simulink model "TV2016"  (Simulink 8.5)
settings: Solver=FixedStepDiscrete  StartTime=0.0  StopTime=inf  FixedStep=0.001  RelTol=1e-3
PreLoadFcn:
  | FSE_Parameters
values from neighbouring files (symbols this model uses):
  car_params = Simulink_Car_params    [TV2016_parameters.m]
  i_Diff = 15.47    [TV2016_parameters.m]
  Kp = 1    [TV2016_parameters.m]
  powerLimitControl = Simulink_el    [TV2016_parameters.m]
  settings = Simulink_Settings    [TV2016_parameters.m]
  SpdC_BCC = 0    [TV2016_parameters.m]
  Speed_Neg_sat = -21    [TV2016_parameters.m]
  Speed_Pos_sat = 21    [TV2016_parameters.m]
  speedEstimation = Simulink_speedEst    [TV2016_parameters.m]
  Tn_n = 0    [TV2016_parameters.m]
  tractionControl = Simulink_tc    [TV2016_parameters.m]
  Use_Joystick = 1    [TV2016_parameters.m]
  yawRateControl = Simulink_yawRate    [TV2016_parameters.m]
libraries: CarMaker4SL x174, simulink x27, simulink_extras x14
(part 3 of 5)

== system TV2016/CarMaker/Control_System /Control /Slip Rate Control  ==
  Ti_ref : Inport
  "States " : Inport  Port=2
  T_req : Inport  Port=3
  Bus Selector : BusSelector  OutputSignals=FL,FR,RL,RR
  Constant : Constant  Value=tractionControl.enable
  Index Vector : MultiPortSwitch  DataPortOrder=Zero-based contiguous  Inputs=2  zeroidx=on
  Mux18 : Mux
  SMC Traction Control : Subsystem  Commented=on
  Traction Controllers : Subsystem
  tcOutput : Scope
      settings: ShowLegends=on  YMin=0.1998305084745763  YMax=0.2840677966101695  SaveName=ScopeData31
  Ti_lim : Outport
  wires:
  "States "/1 -> Traction Controllers/1(states)
  Ti_ref/1 -> Traction Controllers/2(Ti_ref), Index Vector/2
  Index Vector/1 -> Ti_lim/1
  Constant/1 -> Index Vector/1
  T_req/1 -> Traction Controllers/3(T_requested)
  Traction Controllers/1(Ti_SR) -> Bus Selector/1, Index Vector/3
  Mux18/1 -> tcOutput/1
  Bus Selector/1 -> Mux18/1  "<FL>"
  Bus Selector/2 -> Mux18/2  "<FR>"
  Bus Selector/3 -> Mux18/3  "<RL>"
  Bus Selector/4 -> Mux18/4  "<RR>"

== system TV2016/CarMaker/Control_System /Control /Throttle / Brake Mapping ==
  "states " : Inport
  MATLAB Function : MATLAB Function  TreatAsAtomicUnit=on
  T_req : Outport
  wires:
  "states "/1 -> MATLAB Function/1(states)
  MATLAB Function/1(T_req) -> T_req/1

== system TV2016/CarMaker/Control_System /Control /Torque allocation  ==
  Mz_ref : Inport
  T_req : Inport  Port=2
  "States " : Inport  Port=3
  Bus Selector : BusSelector  OutputSignals=mmt_FL,mmt_FR,mmt_RL,mmt_RR
  Index Vector2 : MultiPortSwitch
  MATLAB Function : MATLAB Function  TreatAsAtomicUnit=on
  Mux18 : Mux
  Switch Case : SwitchCase  CaseConditions={1,2,3}
  Switch Case Action Subsystem : Subsystem  TreatAsAtomicUnit=on
  Switch Case Action Subsystem1 : Subsystem  TreatAsAtomicUnit=on
  Switch Case Action Subsystem2 : Subsystem  TreatAsAtomicUnit=on
  Torque Allocation : Subsystem
  maxmotortoruq : Scope
      settings: ShowLegends=on  YMin=0.1998305084745763  YMax=0.2840677966101695  SaveName=ScopeData44
  Ti_lim : Outport
  "Mz_error " : Outport  Port=2
  wires:
  "States "/1 -> MATLAB Function/1(states), Torque Allocation/2(states)
  Mz_ref/1 -> Torque Allocation/4(Mz_ref)
  Torque Allocation/2(Mz_error) -> "Mz_error "/1
  MATLAB Function/1(maxMotorTorque) -> Bus Selector/1, Torque Allocation/3(maxMotorTorque)
  Mux18/1 -> maxmotortoruq/1
  Bus Selector/1 -> Mux18/1  "<mmt_FL>"
  Bus Selector/2 -> Mux18/2  "<mmt_FR>"
  Bus Selector/3 -> Mux18/3  "<mmt_RL>"
  Bus Selector/4 -> Mux18/4  "<mmt_RR>"
  Switch Case/1 -> Switch Case Action Subsystem1/Action
  Switch Case/2 -> Switch Case Action Subsystem/Action
  Switch Case/3 -> Switch Case Action Subsystem2/Action
  ? -> Index Vector2/1, Switch Case/1
  T_req/1 -> Torque Allocation/1(T_req)
  Torque Allocation/1(Ti_lim) -> Ti_lim/1

== system TV2016/CarMaker/Control_System /Control /Yaw Rate Controller  ==
  States : Inport
  "Mz_error " : Inport  Port=2
  Discrete-Time Integrator2 : DiscreteIntegrator  InitialConditionSetting=State (most efficient)  SampleTime=-1
  Enable/disable : Constant  Value=yawRateControl.enable
  Gain : Gain  Gain=single(3.6)
  Gain1 : Gain  Gain=single(3.6)
  Gain2 : Gain  Gain=single(3.6)
  Kd lookup : Lookup_n-D  NumberOfTableDimensions=1  BreakpointsForDimension1="[0  yawRateControl.lookup_speed_end_kmh]"  Table="[yawRateControl.Kd_start  yawRateControl.Kd_end]*yawRateControl.Kd_scaling"  ExtrapMethod=Clip  UseLastTableValue=on  InternalRulePriority=Speed  RndMeth=Simplest  InputSameDT=on
  Ki lookup : Lookup_n-D  NumberOfTableDimensions=1  BreakpointsForDimension1="[0  yawRateControl.lookup_speed_end_kmh]"  Table="[yawRateControl.Ki_start  yawRateControl.Ki_end]*yawRateControl.Ki_scaling"  ExtrapMethod=Clip  UseLastTableValue=on  InternalRulePriority=Speed  RndMeth=Simplest  InputSameDT=on
  Kp Lookup : Lookup_n-D  NumberOfTableDimensions=1  BreakpointsForDimension1="[0  yawRateControl.lookup_speed_end_kmh]"  Table="[yawRateControl.Kp_start  yawRateControl.Kp_end]*yawRateControl.Kp_scaling"  ExtrapMethod=Clip  UseLastTableValue=on  InternalRulePriority=Speed  RndMeth=Simplest  InputSameDT=on
  Ksat : Constant  Value=yawRateControl.Ksat
  "Mzerror " : Scope
      settings: ShowLegends=on  YMin=333.5  YMax=341  SaveName=ScopeData30
  PI_Kp {1..4} (4 alike) : Scope
      PI_Kp 1 settings: ShowLegends=on  YMin=333.5  YMax=341  SaveName=ScopeData3
      PI_Kp 2 settings: ShowLegends=on  YMin=333.5  YMax=341
      PI_Kp 3 settings: ShowLegends=on  TimeRange=4  YMin=333.8411144578313  YMax=336.8411144578313  SaveName=ScopeData9
      PI_Kp 4 settings: ShowLegends=on  YMin=333.5  YMax=341  SaveName=ScopeData18
  Product{7..8,10..11} (4 alike) : Product
  Product3 : Product  OutDataTypeStr=single
  Saturation : Saturate  UpperLimit=yawRateControl.max_moment  LowerLimit=-yawRateControl.max_moment
  Sum2 : Sum  Inputs=+++  AccumDataTypeStr=single
  Sum3 : Sum  Inputs=|+-
  derivative : Scope
      settings: ShowLegends=on  YMin=333.5  YMax=341  SaveName=ScopeData28
  yawRateReference : MATLAB Function  TreatAsAtomicUnit=on
  "r_ref " : Outport
  r_lim : Outport  Port=2
  ay_max : Outport  Port=3
  Mz_ref : Outport  Port=4  OutDataTypeStr=single
  wires:
  States/1 -> yawRateReference/1(states)
  yawRateReference/4(r_ref) -> "r_ref "/1
  yawRateReference/5(r_lim) -> r_lim/1
  yawRateReference/6(ay_max) -> ay_max/1
  Product7/1 -> Sum2/2, PI_Kp 1/1
  Sum2/1 -> Product3/2
  Product8/1 -> Sum3/1
  Sum3/1 -> Discrete-Time Integrator2/1
  Discrete-Time Integrator2/1 -> PI_Kp 3/1, Sum2/3
  Product11/1 -> Sum3/2
  yawRateReference/1(r_der_error) -> Product10/2, PI_Kp 4/1
  Kd lookup/1 -> Product10/1
  Product10/1 -> Sum2/1, derivative/1
  Kp Lookup/1 -> Product7/1
  Ksat/1 -> Product11/1
  "Mz_error "/1 -> "Mzerror "/1, Product11/2
  Ki lookup/1 -> Product8/2
  yawRateReference/2(r_error) -> Product8/1, Product7/2, PI_Kp 2/1
  Product3/1 -> Saturation/1
  Saturation/1 -> Mz_ref/1
  Enable/disable/1 -> Product3/1
  Gain/1 -> Kp Lookup/1
  Gain2/1 -> Ki lookup/1
  yawRateReference/3(vx) -> Gain/1, Gain1/1, Gain2/1
  Gain1/1 -> Kd lookup/1

== system TV2016/CarMaker/IPG Vehicle/Brake/CreateBus Vhcl.Wheel.PT ==
  In : Inport
  BusCreator : BusCreator  Inputs=16
  Demux : Demux  Outputs=16
  Out : Outport
  wires:
  Demux/16 -> BusCreator/16  "Vhcl Wheel RR WhlBearing"
  Demux/15 -> BusCreator/15  "Vhcl Wheel RR Trq_T2W"
  Demux/14 -> BusCreator/14  "Vhcl Wheel RR Trq_BrakeReg_trg"
  Demux/13 -> BusCreator/13  "Vhcl Wheel RR Trq_Brake"
  Demux/12 -> BusCreator/12  "Vhcl Wheel RL WhlBearing"
  Demux/11 -> BusCreator/11  "Vhcl Wheel RL Trq_T2W"
  Demux/10 -> BusCreator/10  "Vhcl Wheel RL Trq_BrakeReg_trg"
  Demux/9 -> BusCreator/9  "Vhcl Wheel RL Trq_Brake"
  Demux/8 -> BusCreator/8  "Vhcl Wheel FR WhlBearing"
  Demux/7 -> BusCreator/7  "Vhcl Wheel FR Trq_T2W"
  Demux/6 -> BusCreator/6  "Vhcl Wheel FR Trq_BrakeReg_trg"
  Demux/5 -> BusCreator/5  "Vhcl Wheel FR Trq_Brake"
  Demux/4 -> BusCreator/4  "Vhcl Wheel FL WhlBearing"
  Demux/3 -> BusCreator/3  "Vhcl Wheel FL Trq_T2W"
  Demux/2 -> BusCreator/2  "Vhcl Wheel FL Trq_BrakeReg_trg"
  Demux/1 -> BusCreator/1  "Vhcl Wheel FL Trq_Brake"
  BusCreator/1 -> Out/1
  In/1 -> Demux/1

== system TV2016/CarMaker/IPG Vehicle/CarAndTrailer/CarAndTrailerUpd ==
  Sync_In : Inport
  Vhcl.Steering : Inport  Port=2
  Vhcl.Motion : Inport  Port=3
  Vhcl.PoI : Inport  Port=4
  Vhcl.Wheel.FL : Inport  Port=5
  Vhcl.Wheel.FR : Inport  Port=6
  Vhcl.Wheel.RL : Inport  Port=7
  Vhcl.Wheel.RR : Inport  Port=8
  Car.Hitch.FrcTrq : Inport  Port=9
  Vhcl.Fr1A : Inport  Port=10
  CarAndTrailerUpd : S-Function  FunctionName=CM_Sfun  Parameters='CarAndTrUpd'
  CreateBus Brake.IF.In : Subsystem
  Sync_Out : Outport
  Brake.IF.In : Outport  Port=2
  wires:
  Vhcl.Fr1A/1 -> CarAndTrailerUpd/10  "user vehicle only"
  Vhcl.Steering/1 -> CarAndTrailerUpd/2
  Vhcl.Motion/1 -> CarAndTrailerUpd/3
  Vhcl.PoI/1 -> CarAndTrailerUpd/4
  Vhcl.Wheel.FL/1 -> CarAndTrailerUpd/5
  Vhcl.Wheel.FR/1 -> CarAndTrailerUpd/6
  Car.Hitch.FrcTrq/1 -> CarAndTrailerUpd/9
  Vhcl.Wheel.RR/1 -> CarAndTrailerUpd/8
  Vhcl.Wheel.RL/1 -> CarAndTrailerUpd/7
  CarAndTrailerUpd/2 -> CreateBus Brake.IF.In/1(In)
  CreateBus Brake.IF.In/1(Out) -> Brake.IF.In/1
  CarAndTrailerUpd/1 -> Sync_Out/1
  Sync_In/1 -> CarAndTrailerUpd/1

== system TV2016/CarMaker/IPG Vehicle/CarAndTrailer/Forces ==
  Sync_In : Inport
  TireFL_In : Inport  Port=2
  TireFR_In : Inport  Port=3
  TireRL_In : Inport  Port=4
  TireRR_In : Inport  Port=5
  lSpring : Inport  Port=6
  vDamp : Inport  Port=7
  lStabi : Inport  Port=8
  lBuf : Inport  Port=9
  External Suspension Forces : Subsystem
  Tires : Subsystem
  Vehicle Forces : Subsystem
  Sync_Out : Outport
  Car.Virtual : Outport  Port=2
  Car.Aero : Outport  Port=3
  Car.Load : Outport  Port=4
  TireFL_Out : Outport  Port=5
  TireFR_Out : Outport  Port=6
  TireRL_Out : Outport  Port=7
  TireRR_Out : Outport  Port=8
  FSpring : Outport  Port=9
  FDamp : Outport  Port=10
  FStabi : Outport  Port=11
  FBuf : Outport  Port=12
  wires:
  External Suspension Forces/4(FBuf) -> FBuf/1
  lBuf/1 -> External Suspension Forces/5(lBuf)
  Tires/1(TireFL_Out) -> TireFL_Out/1
  Tires/4(TireRR_Out) -> TireRR_Out/1
  Tires/3(TireRL_Out) -> TireRL_Out/1
  Tires/2(TireFR_Out) -> TireFR_Out/1
  TireRR_In/1 -> Tires/4(TireRR_In)
  TireRL_In/1 -> Tires/3(TireRL_In)
  TireFR_In/1 -> Tires/2(TireFR_In)
  Sync_In/1 -> External Suspension Forces/1(Sync_In), Tires/5(Sync_In), Vehicle Forces/1(Sync_In)
  Vehicle Forces/1(Sync_Out) -> Sync_Out/1
  TireFL_In/1 -> Tires/1(TireFL_In)
  Vehicle Forces/2(Car.Virtual) -> Car.Virtual/1
  Vehicle Forces/3(Car.Aero) -> Car.Aero/1
  Vehicle Forces/4(Car.Load) -> Car.Load/1
  lSpring/1 -> External Suspension Forces/2(lSpring)
  External Suspension Forces/2(FDamp) -> FDamp/1
  vDamp/1 -> External Suspension Forces/3(vDamp)
  lStabi/1 -> External Suspension Forces/4(lStabi)
  External Suspension Forces/3(FStabi) -> FStabi/1
  External Suspension Forces/1(FSpring) -> FSpring/1

== system TV2016/CarMaker/IPG Vehicle/CarAndTrailer/Kinematics ==
  Sync_In : Inport
  Steer.IF : Inport  Port=2
  Kinematics : S-Function  FunctionName=CM_Sfun  Parameters='Kinematics'
  Sync_Out : Outport
  TireFL_In : Outport  Port=2
  TireFR_In : Outport  Port=3
  TireRL_In : Outport  Port=4
  TireRR_In : Outport  Port=5
  lSpring : Outport  Port=6
  vDamp : Outport  Port=7
  lStabi : Outport  Port=8
  lBuf : Outport  Port=9
  wires:
  Kinematics/9 -> lBuf/1
  Kinematics/8 -> lStabi/1
  Kinematics/2 -> TireFL_In/1
  Kinematics/3 -> TireFR_In/1
  Kinematics/4 -> TireRL_In/1
  Kinematics/5 -> TireRR_In/1
  Kinematics/6 -> lSpring/1
  Kinematics/7 -> vDamp/1
  Sync_In/1 -> Kinematics/1
  Kinematics/1 -> Sync_Out/1
  Steer.IF/1 -> Kinematics/2

== system TV2016/CarMaker/IPG Vehicle/CarAndTrailer/Kinetics ==
  Sync_In : Inport
  Car.Virtual : Inport  Port=2
  Car.Aero : Inport  Port=3
  Car.Load : Inport  Port=4
  TireFL.Out : Inport  Port=5
  TireFR.Out : Inport  Port=6
  TireRL.Out : Inport  Port=7
  TireRR.Out : Inport  Port=8
  FSpring : Inport  Port=9
  FDamp : Inport  Port=10
  FStabi : Inport  Port=11
  FBuf : Inport  Port=12
  Bus Creator : BusCreator
  Bus Creator1 : BusCreator  Inputs=12
  Bus Creator2 : BusCreator  Inputs=6
  Bus Creator3 : BusCreator  Inputs=6
  Bus Creator4 : BusCreator
  Demux : Demux  Outputs=12
  Demux1 : Demux  Outputs=6
  Demux2 : Demux  Outputs=6
  Demux3 : Demux
  Demux4 : Demux
  Kinetics : S-Function  FunctionName=CM_Sfun  Parameters='Kinetics'
  Sync_Out : Outport
  Trailer.Load : Outport  Port=2
  Car.Hitch : Outport  Port=3
  Car.Fr1 : Outport  Port=4
  Car.Trq_T2W : Outport  Port=5
  WheelCarrier.Misc : Outport  Port=6
  wires:
  FBuf/1 -> Kinetics/12
  Sync_In/1 -> Kinetics/1
  Kinetics/1 -> Sync_Out/1
  Car.Aero/1 -> Kinetics/3
  Car.Virtual/1 -> Kinetics/2
  Bus Creator1/1 -> Trailer.Load/1
  Demux/1 -> Bus Creator1/1  "Trailer Load_0 mass"
  Demux/2 -> Bus Creator1/2  "Trailer Load_0 tx"
  Demux/3 -> Bus Creator1/3  "Trailer Load_0 ty"
  Demux/4 -> Bus Creator1/4  "Trailer Load_0 tz"
  Kinetics/2 -> Demux/1
  Demux/5 -> Bus Creator1/5  "Trailer Load_1 mass"
  Demux/6 -> Bus Creator1/6  "Trailer Load_1 tx"
  Demux/7 -> Bus Creator1/7  "Trailer Load_1 ty"
  Demux/8 -> Bus Creator1/8  "Trailer Load_1 tz"
  Demux/9 -> Bus Creator1/9  "Trailer Load_2 mass"
  Demux/10 -> Bus Creator1/10  "Trailer Load_2 tx"
  Demux/11 -> Bus Creator1/11  "Trailer Load_2 ty"
  Demux/12 -> Bus Creator1/12  "Trailer Load_2 tz"
  Demux1/1 -> Bus Creator2/1  "Car Hitch tx"
  Demux1/2 -> Bus Creator2/2  "Car Hitch ty"
  Demux1/3 -> Bus Creator2/3  "Car Hitch tz"
  Demux1/4 -> Bus Creator2/4  "Car Hitch vx"
  Demux1/5 -> Bus Creator2/5  "Car Hitch vy"
  Demux1/6 -> Bus Creator2/6  "Car Hitch vz"
  Kinetics/3 -> Demux1/1
  Bus Creator2/1 -> Car.Hitch/1
  Demux2/1 -> Bus Creator3/1  "Car Fr1 rx"
  Demux2/2 -> Bus Creator3/2  "Car Fr1 ry"
  Demux2/3 -> Bus Creator3/3  "Car Fr1 rz"
  Demux2/4 -> Bus Creator3/4  "Car Fr1 rvx"
  Demux2/5 -> Bus Creator3/5  "Car Fr1 rvy"
  Demux2/6 -> Bus Creator3/6  "Car Fr1 rvz"
  Bus Creator3/1 -> Car.Fr1/1
  Kinetics/4 -> Demux2/1
  Car.Load/1 -> Kinetics/4
  Demux3/1 -> Bus Creator4/1  "car Susp FL GenInert2"
  Demux3/2 -> Bus Creator4/2  "car Susp FR GenInert2"
  Demux3/3 -> Bus Creator4/3  "car Susp FL GenFrc2"
  Demux3/4 -> Bus Creator4/4  "car Susp FR GenFrc2"
  Bus Creator4/1 -> WheelCarrier.Misc/1
  Bus Creator/1 -> Car.Trq_T2W/1
  Demux4/4 -> Bus Creator/4  "Car Trq_T2WRR"
  Demux4/3 -> Bus Creator/3  "Car Trq_T2WRL"
  Demux4/2 -> Bus Creator/2  "Car Trq_T2WFR"
  Demux4/1 -> Bus Creator/1  "Car Trq_T2WFL"
  TireFL.Out/1 -> Kinetics/5
  TireFR.Out/1 -> Kinetics/6
  TireRL.Out/1 -> Kinetics/7
  TireRR.Out/1 -> Kinetics/8
  FSpring/1 -> Kinetics/9
  FDamp/1 -> Kinetics/10
  FStabi/1 -> Kinetics/11
  Kinetics/6 -> Demux3/1
  Kinetics/5 -> Demux4/1

== system TV2016/CarMaker/IPG Vehicle/CarAndTrailer/Steering ==
  note: When replacing the entire steering system,
      | be sure to add '-disablesteering' to the command line arguments
      | in the CarMaker Model Configuration block.
  Sync_In : Inport
  VhclCtrl.Steering : Inport  Port=2
  Bus Creator1 : BusCreator  Inputs=16
  Bus Creator2 : BusCreator
  Demux : Demux  Outputs=20
  Steering : S-Function  FunctionName=CM_Sfun  Parameters='Steering'
  Terminator : Terminator
  Sync_Out : Outport
  Steer.IF : Outport  Port=2
  wires:
  Bus Creator1/1 -> Steer.IF/1
  Steering/2 -> Demux/1
  Demux/8 -> Bus Creator1/8  "Steering IF AssistTrqPin"
  Demux/7 -> Bus Creator1/7  "Steering IF AssistTrqCol"
  Demux/6 -> Bus Creator1/6  "Steering IF AssistFrc"
  Demux/20 -> Bus Creator2/4  "Steering IF R Inert"
  Demux/17 -> Bus Creator2/1  "Steering IF L Frc"
  Demux/18 -> Bus Creator2/2  "Steering IF L Inert"
  Demux/19 -> Bus Creator2/3  "Steering IF R Frc"
  Bus Creator2/1 -> Terminator/1  "Steer IF (in)"
  Demux/16 -> Bus Creator1/16  "Steering IF R iSteer2q"
  Demux/9 -> Bus Creator1/9  "Steering IF L q"
  Demux/10 -> Bus Creator1/10  "Steering IF L qp"
  Demux/11 -> Bus Creator1/11  "Steering IF L qpp"
  Demux/12 -> Bus Creator1/12  "Steering IF L iSteer2q"
  Demux/13 -> Bus Creator1/13  "Steering IF R q"
  Demux/14 -> Bus Creator1/14  "Steering IF R qp"
  Demux/15 -> Bus Creator1/15  "Steering IF R qpp"
  VhclCtrl.Steering/1 -> Steering/2
  Steering/1 -> Sync_Out/1
  Sync_In/1 -> Steering/1
  Demux/1 -> Bus Creator1/1  "Steering IF Ang"
  Demux/2 -> Bus Creator1/2  "Steering IF AngVel"
  Demux/3 -> Bus Creator1/3  "Steering IF AngAcc"
  Demux/4 -> Bus Creator1/4  "Steering IF Trq"
  Demux/5 -> Bus Creator1/5  "Steering IF TrqStatic"

== system TV2016/CarMaker/IPG Vehicle/CarAndTrailer/Trailer ==
  Sync_In : Inport
  Trailer.Load : Inport  Port=2
  Car.Hitch : Inport  Port=3
  Car.Fr1 : Inport  Port=4
  Car.Trq_T2W : Inport  Port=5
  WheelCarrier.Misc : Inport  Port=6
  CreateBus Car.Hitch.FrcTrq : Subsystem
  CreateBus Vhcl.Motion : Subsystem
  CreateBus Vhcl.PoI : Subsystem
  CreateBus Vhcl.Steering : Subsystem
  CreateBus Vhcl.Wheel.FL : Subsystem
  CreateBus Vhcl.Wheel.FR : Subsystem
  CreateBus Vhcl.Wheel.RL : Subsystem
  CreateBus Vhcl.Wheel.RR : Subsystem
  Trailer : S-Function  FunctionName=CM_Sfun  Parameters='Trailer'
  Sync_Out : Outport
  Vhcl.Steering : Outport  Port=2
  Vhcl.Motion : Outport  Port=3
  Vhcl.PoI : Outport  Port=4
  Vhcl.Wheel.FL : Outport  Port=5
  Vhcl.Wheel.FR : Outport  Port=6
  Vhcl.Wheel.RL : Outport  Port=7
  Vhcl.Wheel.RR : Outport  Port=8
  Car.Hitch.FrcTrq : Outport  Port=9
  wires:
  Trailer/2 -> CreateBus Vhcl.Steering/1(In1)
  CreateBus Vhcl.Steering/1(Out1) -> Vhcl.Steering/1
  Trailer/3 -> CreateBus Vhcl.Motion/1(In1)
  Trailer/4 -> CreateBus Vhcl.PoI/1(In1)
  Trailer/5 -> CreateBus Vhcl.Wheel.FL/1(In1)
  Trailer/6 -> CreateBus Vhcl.Wheel.FR/1(In1)
  Trailer/7 -> CreateBus Vhcl.Wheel.RL/1(In1)
  Trailer/9 -> CreateBus Car.Hitch.FrcTrq/1(In1)
  Trailer/8 -> CreateBus Vhcl.Wheel.RR/1(In1)
  CreateBus Vhcl.Wheel.RR/1(Out1) -> Vhcl.Wheel.RR/1  "Vhcl.Wheel.RR"
  CreateBus Vhcl.Wheel.RL/1(Out1) -> Vhcl.Wheel.RL/1  "Vhcl.Wheel.RL"
  CreateBus Vhcl.Wheel.FR/1(Out1) -> Vhcl.Wheel.FR/1  "Vhcl.Wheel.FR"
  CreateBus Vhcl.Wheel.FL/1(Out1) -> Vhcl.Wheel.FL/1  "Vhcl.Wheel.FL"
  CreateBus Vhcl.PoI/1(Out1) -> Vhcl.PoI/1
  CreateBus Vhcl.Motion/1(Out1) -> Vhcl.Motion/1
  Car.Trq_T2W/1 -> Trailer/5
  WheelCarrier.Misc/1 -> Trailer/6
  CreateBus Car.Hitch.FrcTrq/1(Car.Hitch.FrcTrq) -> Car.Hitch.FrcTrq/1
  Car.Fr1/1 -> Trailer/4
  Car.Hitch/1 -> Trailer/3
  Trailer.Load/1 -> Trailer/2
  Trailer/1 -> Sync_Out/1
  Sync_In/1 -> Trailer/1

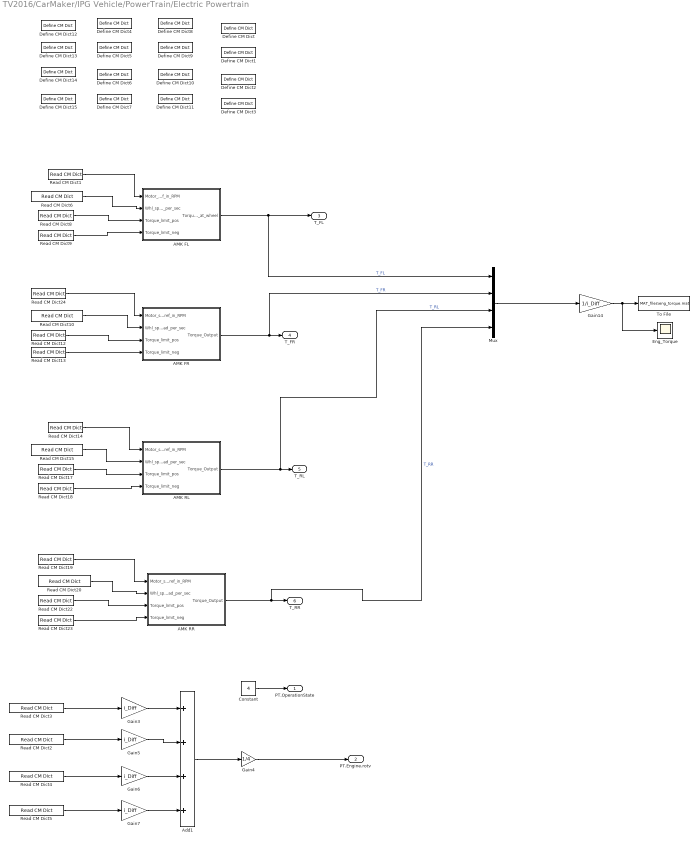
== system TV2016/CarMaker/IPG Vehicle/PowerTrain/Electric Powertrain ==
  AMK FL : Subsystem
  AMK FR : Subsystem
  AMK RL : Subsystem
  AMK RR : Subsystem
  Add1 : Sum  Inputs=++++
  Constant : Constant  Value=4
  Define CM Dict : CarMaker4SL/Define CM Dict  xname=T_req_RL  xmono=off  xtype=Double4  xdvaplace=None  xnstates=0  xfirststate=0  xinitial=0
  Define CM Dict1 : CarMaker4SL/Define CM Dict  xname=T_req_RR  xmono=off  xtype=Double4  xdvaplace=None  xnstates=0  xfirststate=0  xinitial=0
  Define CM Dict10 : CarMaker4SL/Define CM Dict  xname=Tlim_neg_RL  xmono=off  xtype=Double4  xdvaplace=None  xnstates=0  xfirststate=0  xinitial=0
  Define CM Dict11 : CarMaker4SL/Define CM Dict  xname=Tlim_neg_RR  xmono=off  xtype=Double4  xdvaplace=None  xnstates=0  xfirststate=0  xinitial=0
  Define CM Dict12 : CarMaker4SL/Define CM Dict  xname=w_set_FL  xmono=off  xtype=Double4  xdvaplace=None  xnstates=0  xfirststate=0  xinitial=0
  Define CM Dict13 : CarMaker4SL/Define CM Dict  xname=w_set_FR  xmono=off  xtype=Double4  xdvaplace=None  xnstates=0  xfirststate=0  xinitial=0
  Define CM Dict14 : CarMaker4SL/Define CM Dict  xname=w_set_RL  xmono=off  xtype=Double4  xdvaplace=None  xnstates=0  xfirststate=0  xinitial=0
  Define CM Dict15 : CarMaker4SL/Define CM Dict  xname=w_set_RR  xmono=off  xtype=Double4  xdvaplace=None  xnstates=0  xfirststate=0  xinitial=0
  Define CM Dict2 : CarMaker4SL/Define CM Dict  xname=T_req_FL  xmono=off  xtype=Double4  xdvaplace=None  xnstates=0  xfirststate=0  xinitial=0
  Define CM Dict3 : CarMaker4SL/Define CM Dict  xname=T_req_FR  xmono=off  xtype=Double4  xdvaplace=None  xnstates=0  xfirststate=0  xinitial=0
  Define CM Dict4 : CarMaker4SL/Define CM Dict  xname=Tlim_pos_FL  xmono=off  xtype=Double4  xdvaplace=None  xnstates=0  xfirststate=0  xinitial=0
  Define CM Dict5 : CarMaker4SL/Define CM Dict  xname=Tlim_pos_FR  xmono=off  xtype=Double4  xdvaplace=None  xnstates=0  xfirststate=0  xinitial=0
  Define CM Dict6 : CarMaker4SL/Define CM Dict  xname=Tlim_pos_RL  xmono=off  xtype=Double4  xdvaplace=None  xnstates=0  xfirststate=0  xinitial=0
  Define CM Dict7 : CarMaker4SL/Define CM Dict  xname=Tlim_pos_RR  xmono=off  xtype=Double4  xdvaplace=None  xnstates=0  xfirststate=0  xinitial=0
  Define CM Dict8 : CarMaker4SL/Define CM Dict  xname=Tlim_neg_FL  xmono=off  xtype=Double4  xdvaplace=None  xnstates=0  xfirststate=0  xinitial=0
  Define CM Dict9 : CarMaker4SL/Define CM Dict  xname=Tlim_neg_FR  xmono=off  xtype=Double4  xdvaplace=None  xnstates=0  xfirststate=0  xinitial=0
  "Eng_Torque " : Scope
      settings: ShowLegends=on  TimeRange=0.934067321532285  YMin=7.026767000833312  YMax=8.703492336052118  SaveName=ScopeData23
  Gain14 : Gain  Gain=1/i_Diff
  Gain{3,5..7} (4 alike) : Gain  Gain=i_Diff
  Gain4 : Gain  Gain=1/4
  Mux : Mux
  Read CM Dict1 : CarMaker4SL/Read CM Dict  xname=w_set_FL  xsync=off
  Read CM Dict10 : CarMaker4SL/Read CM Dict  xname=Car.WheelSpd_FR  xsync=off
  Read CM Dict12 : CarMaker4SL/Read CM Dict  xname=Tlim_pos_FR  xsync=off
  Read CM Dict13 : CarMaker4SL/Read CM Dict  xname=Tlim_neg_FR  xsync=off
  Read CM Dict14 : CarMaker4SL/Read CM Dict  xname=w_set_RL  xsync=off
  Read CM Dict15 : CarMaker4SL/Read CM Dict  xname=Car.WheelSpd_RL  xsync=off
  Read CM Dict17 : CarMaker4SL/Read CM Dict  xname=Tlim_pos_RL  xsync=off
  Read CM Dict18 : CarMaker4SL/Read CM Dict  xname=Tlim_neg_RL  xsync=off
  Read CM Dict19 : CarMaker4SL/Read CM Dict  xname=w_set_RR  xsync=off
  Read CM Dict2 : CarMaker4SL/Read CM Dict  xname=Car.WheelSpd_RR  xsync=off
  Read CM Dict20 : CarMaker4SL/Read CM Dict  xname=Car.WheelSpd_RR  xsync=off
  Read CM Dict22 : CarMaker4SL/Read CM Dict  xname=Tlim_pos_RR  xsync=off
  Read CM Dict23 : CarMaker4SL/Read CM Dict  xname=Tlim_neg_RR  xsync=off
  Read CM Dict24 : CarMaker4SL/Read CM Dict  xname=w_set_FR  xsync=off
  Read CM Dict3 : CarMaker4SL/Read CM Dict  xname=Car.WheelSpd_RL  xsync=off
  Read CM Dict4 : CarMaker4SL/Read CM Dict  xname=Car.WheelSpd_FR  xsync=off
  Read CM Dict5 : CarMaker4SL/Read CM Dict  xname=Car.WheelSpd_FL  xsync=off
  Read CM Dict6 : CarMaker4SL/Read CM Dict  xname=Car.WheelSpd_FL  xsync=off
  Read CM Dict8 : CarMaker4SL/Read CM Dict  xname=Tlim_pos_FL  xsync=off
  Read CM Dict9 : CarMaker4SL/Read CM Dict  xname=Tlim_neg_FL  xsync=off
  To File : ToFile  Filename=MAT_files\eng_torque.mat  MatrixName=torques  SaveFormat=Timeseries
  PT.OperationState : Outport
  PT.Engine.rotv : Outport  Port=2
  T_FL : Outport  Port=3
  T_FR : Outport  Port=4
  T_RL : Outport  Port=5
  T_RR : Outport  Port=6
  wires:
  Constant/1 -> PT.OperationState/1
  Gain3/1 -> Add1/1
  Gain5/1 -> Add1/2
  Add1/1 -> Gain4/1
  Gain4/1 -> PT.Engine.rotv/1
  Gain6/1 -> Add1/3
  Gain7/1 -> Add1/4
  Read CM Dict6/1 -> AMK FL/2(Whl_speed_rad_per_sec)
  Read CM Dict9/1 -> AMK FL/4(Torque_limit_neg)
  Read CM Dict1/1 -> AMK FL/1(Motor_speed_ref_in_RPM)
  AMK FL/1("Torque_output_at_wheel ") -> T_FL/1, Mux/1  "T_FL"
  Read CM Dict10/1 -> AMK FR/2(Whl_speed_rad_per_sec)
  Read CM Dict12/1 -> AMK FR/3("Torque_limit_pos ")
  Read CM Dict13/1 -> AMK FR/4(Torque_limit_neg)
  Read CM Dict24/1 -> AMK FR/1(Motor_speed_ref_in_RPM)
  AMK FR/1("Torque_Output ") -> Mux/2, T_FR/1  "T_FR"
  Read CM Dict17/1 -> AMK RL/3("Torque_limit_pos ")
  Read CM Dict18/1 -> AMK RL/4(Torque_limit_neg)
  Read CM Dict14/1 -> AMK RL/1(Motor_speed_ref_in_RPM)
  AMK RL/1("Torque_Output ") -> Mux/3, T_RL/1  "T_RL"
  Read CM Dict20/1 -> AMK RR/2(Whl_speed_rad_per_sec)
  Read CM Dict22/1 -> AMK RR/3("Torque_limit_pos ")
  Read CM Dict23/1 -> AMK RR/4(Torque_limit_neg)
  Read CM Dict19/1 -> AMK RR/1(Motor_speed_ref_in_RPM)
  AMK RR/1("Torque_Output ") -> T_RR/1, Mux/4  "T_RR"
  Mux/1 -> Gain14/1
  Gain14/1 -> "Eng_Torque "/1, To File/1
  Read CM Dict3/1 -> Gain3/1
  Read CM Dict2/1 -> Gain5/1
  Read CM Dict4/1 -> Gain6/1
  Read CM Dict5/1 -> Gain7/1
  Read CM Dict8/1 -> AMK FL/3("Torque_limit_pos ")
  Read CM Dict15/1 -> AMK RL/2(Whl_speed_rad_per_sec)

== system TV2016/CarMaker/VehicleControl/CreateBus VhclCtrl/RacingwheelInterface ==
  Add KERS : MATLAB Function  TreatAsAtomicUnit=on
  Constant1 : Constant  Value=-1
  Constant2 : Constant  Value=0.5
  Constant4 : Constant
  Constant5 : Constant  Value=-1
  Constant6 : Constant
  Data Type Conversion1 : DataTypeConversion  OutDataTypeStr=double
  Demux : Demux  Outputs=5
  Gain : Gain  Gain=0.3
  Gain1 : Gain  Gain=0.3
  Product{,1,3..4} (4 alike) : Product
  Saturation : Saturate  UpperLimit=0.95  LowerLimit=0
  Sum1 : Sum  Inputs=|++
  Sum3 : Sum  Inputs=|++
  "Vx " : Scope
      settings: TimeRange=6  YMin=-2  YMax=12  SaveName=ScopeData56
  Vx 1 : Scope
      settings: TimeRange=6  YMin=-2  YMax=12  SaveName=ScopeData10
  Vx 4 : Scope
      settings: TimeRange=6  YMin=-2  YMax=12  SaveName=ScopeData60
  brake : Scope
      settings: TimeRange=6  YMin=-1  YMax=1  SaveName=ScopeData59
  steering : Scope
      settings: TimeRange=6  YMin=-2  YMax=12  SaveName=ScopeData66
  throttle : Scope
      settings: TimeRange=6  YMin=-2  YMax=12  SaveName=ScopeData62
  "Steering " : Outport
  throttleinoput : Outport  Port=2
  brake input : Outport  Port=3
  wires:
  ? -> "Vx "/1, Demux/1
  Demux/4 -> Vx 4/1
  Demux/1 -> Product/1  "steering"
  Constant1/1 -> Product/2
  Constant2/1 -> Product1/2
  Product/1 -> steering/1, "Steering "/1
  Product1/1 -> Saturation/1
  Constant4/1 -> Sum1/2
  Sum1/1 -> Product1/1
  Demux/2 -> Product3/1  "throttle"
  Constant5/1 -> Product3/2, Product4/2
  Product3/1 -> Sum1/1
  Constant6/1 -> Sum3/2
  Sum3/1 -> Gain/1
  Product4/1 -> Sum3/1
  Demux/3 -> Product4/1  "brake"
  ? -> Vx 1/1
  Saturation/1 -> throttle/1, throttleinoput/1
  Add KERS/1(KERS_pos) -> brake/1, Data Type Conversion1/1
  Data Type Conversion1/1 -> ?
  Add KERS/2(brake_pos) -> brake input/1
  Gain/1 -> Add KERS/1(brake_pedal)

== system TV2016/CarMaker/Control_System /Control /Slip Rate Control /SMC Traction Control ==
  note: Tc ouput is either an increase or decrease in torque .
  states : Inport
  Ti_ref : Inport  Port=2
  T_requested : Inport  Port=3
  Bus Selector : BusSelector  OutputSignals=FL,FR,RL,RR
  Constant : Constant  Value=tractionControl.Kp
  Constant1 : Constant  Value=tractionControl.Ki
  Constant2 : Constant  Value=tractionControl.Slip_ratio_ref
  Gain : Gain  Gain=single(3.6)
  Gain2 : Gain  Gain=single(3.6)
  Ki Loopup : Lookup_n-D  NumberOfTableDimensions=1  BreakpointsForDimension1=[0 5 10]  Table="[tractionControl.Ki_start tractionControl.Ki_middle  tractionControl.Ki_end]*tractionControl.Ki_scaling"  ExtrapMethod=Clip  UseLastTableValue=on  InternalRulePriority=Speed  RndMeth=Simplest  InputSameDT=on
  Kp Lookup : Lookup_n-D  NumberOfTableDimensions=1  BreakpointsForDimension1="[0  5]"  Table="[tractionControl.Kp_start  tractionControl.Kp_end]*tractionControl.Kp_scaling"  ExtrapMethod=Clip  UseLastTableValue=on  InternalRulePriority=Speed  RndMeth=Simplest  InputSameDT=on
  MATLAB Function : MATLAB Function  TreatAsAtomicUnit=on
  MATLAB Function1 : MATLAB Function  TreatAsAtomicUnit=on
  Slip Rate FL : Subsystem
  Slip Rate FL1 : Subsystem
  Slip Rate FL2 : Subsystem
  Slip Rate FL3 : Subsystem
  Ti_SR : Outport
  wires:
  states/1 -> MATLAB Function1/1(states), Slip Rate FL/4(states), Slip Rate FL1/4(states), Slip Rate FL2/4(states), Slip Rate FL3/4(states), MATLAB Function/9(states)
  Ti_ref/1 -> Bus Selector/1
  Bus Selector/1 -> [Ti_FL]  "<FL>"
  Bus Selector/2 -> [Ti_FR]  "<FR>"
  Bus Selector/3 -> [Ti_RL]  "<RL>"
  Bus Selector/4 -> [Ti_RR]  "<RR>"
  [SR_Kp] -> Slip Rate FL/2(Kp)
  Kp Lookup/1 -> ?
  Ki Loopup/1 -> [SR_Ki]
  Gain/1 -> Kp Lookup/1
  Gain2/1 -> Ki Loopup/1
  Constant1/1 -> ?
  Constant/1 -> [SR_Kp]
  MATLAB Function/1(Ti_lim) -> Ti_SR/1
  [Ti_FL] -> MATLAB Function/1(Ti_FL)
  [Ti_RR] -> MATLAB Function/4(Ti_RR)
  [Ti_RL] -> MATLAB Function/3(Ti_RL)
  [Ti_FR] -> MATLAB Function/2(Ti_FR)
  T_requested/1 -> MATLAB Function/10(T_req)
  MATLAB Function1/1(SR_FL) -> Slip Rate FL/3(SR)
  Constant2/1 -> Slip Rate FL3/1(SR_ref), Slip Rate FL2/1(SR_ref), Slip Rate FL1/1(SR_ref), Slip Rate FL/1(SR_ref)
  MATLAB Function1/5(vx) -> Gain2/1, Gain/1
  MATLAB Function1/2(SR_FR) -> Slip Rate FL1/3(SR)
  MATLAB Function1/3(SR_RL) -> Slip Rate FL2/3(SR)
  MATLAB Function1/4(SR_RR) -> Slip Rate FL3/3(SR)
  [SR_Kp] -> Slip Rate FL1/2(Kp)
  [SR_Kp] -> Slip Rate FL2/2(Kp)
  [SR_Kp] -> Slip Rate FL3/2(Kp)
  Slip Rate FL/1(Tc) -> MATLAB Function/5(TC_FL)
  Slip Rate FL1/1(Tc) -> MATLAB Function/6(TC_FR)
  Slip Rate FL2/1(Tc) -> MATLAB Function/7(TC_RL)
  Slip Rate FL3/1(Tc) -> MATLAB Function/8(TC_RR)

== system TV2016/CarMaker/Control_System /Control /Slip Rate Control /Traction Controllers ==
  states : Inport
  Ti_ref : Inport  Port=2
  T_requested : Inport  Port=3
  Bus Selector : BusSelector  OutputSignals=FL,FR,RL,RR
  Constant2 : Constant  Value=tractionControl.Slip_ratio_ref
  MATLAB Function : MATLAB Function  TreatAsAtomicUnit=on
  MATLAB Function1 : MATLAB Function  TreatAsAtomicUnit=on
  Mux18 : Mux
  Slip Rate FL : Subsystem
  Slip Rate FR : Subsystem
  Slip Rate RL : Subsystem
  Slip Rate RR : Subsystem
  tcOutput : Scope
      settings: ShowLegends=on  YMin=0.1998305084745763  YMax=0.2840677966101695  SaveName=ScopeData43
  Ti_SR : Outport
  wires:
  states/1 -> MATLAB Function1/1(states), MATLAB Function/9(states)
  Ti_ref/1 -> MATLAB Function1/3(T_tv), Bus Selector/1
  Bus Selector/1 -> [Ti_FL]  "<FL>"
  Bus Selector/2 -> [Ti_FR]  "<FR>"
  Bus Selector/3 -> [Ti_RL]  "<RL>"
  Bus Selector/4 -> [Ti_RR]  "<RR>"
  [Ti_FL] -> Slip Rate FL/5(Ti_ref)
  [Ti_FR] -> Slip Rate FR/5(Ti_ref)
  [Ti_RL] -> Slip Rate RL/5(Ti_ref)
  [Ti_RR] -> Slip Rate RR/5(Ti_ref)
  [SR_Ki] -> Slip Rate FL/3(Ki)
  [SR_Kp] -> Slip Rate FL/2(Kp)
  [SR_Kp] -> Slip Rate FR/2(Kp)
  [SR_Ki] -> Slip Rate FR/3(Ki)
  [SR_Kp] -> Slip Rate RL/2(Kp)
  [SR_Ki] -> Slip Rate RL/3(Ki)
  [SR_Kp] -> Slip Rate RR/2(Kp)
  [SR_Ki] -> Slip Rate RR/3(Ki)
  Slip Rate FL/1(TC_output) -> Mux18/1, MATLAB Function/5(TC_FL)  "FL"
  Slip Rate FR/1(TC_output) -> Mux18/2, MATLAB Function/6(TC_FR)  "FR"
  Slip Rate RR/1(TC_output) -> Mux18/4, MATLAB Function/8(TC_RR)  "RR"
  Slip Rate RL/1(TC_output) -> Mux18/3, MATLAB Function/7(TC_RL)  "RL"
  MATLAB Function/1(Ti_lim) -> Ti_SR/1
  [Ti_FL] -> MATLAB Function/1(Ti_FL)
  [Ti_RR] -> MATLAB Function/4(Ti_RR)
  [Ti_RL] -> MATLAB Function/3(Ti_RL)
  [Ti_FR] -> MATLAB Function/2(Ti_FR)
  T_requested/1 -> MATLAB Function1/2(T_req), MATLAB Function/10(T_req)
  MATLAB Function1/2(SR_FR) -> Slip Rate FR/4(SR)
  MATLAB Function1/3(SR_RL) -> Slip Rate RL/4(SR)
  Constant2/1 -> Slip Rate RR/1(SR_ref), Slip Rate RL/1(SR_ref), Slip Rate FR/1(SR_ref), Slip Rate FL/1(SR_ref)
  MATLAB Function1/4(SR_RR) -> Slip Rate RR/4(SR)
  MATLAB Function1/1(SR_FL) -> Slip Rate FL/4(SR)
  MATLAB Function1/5(Kp) -> [SR_Kp]
  MATLAB Function1/6(Ki) -> [SR_Ki]
  Mux18/1 -> tcOutput/1

== system TV2016/CarMaker/Control_System /Control /Torque allocation /Switch Case Action Subsystem ==
  In1 : Inport
  Action Port : ActionPort  ActionType=case
  Out1 : Outport
  wires:
  In1/1 -> Out1/1

== system TV2016/CarMaker/Control_System /Control /Torque allocation /Switch Case Action Subsystem1 ==
  In1 : Inport
  Action Port : ActionPort  ActionType=case
  Out1 : Outport
  wires:
  In1/1 -> Out1/1

== system TV2016/CarMaker/Control_System /Control /Torque allocation /Switch Case Action Subsystem2 ==
  In1 : Inport
  Action Port : ActionPort  ActionType=case
  Out1 : Outport
  wires:
  In1/1 -> Out1/1

== system TV2016/CarMaker/Control_System /Control /Torque allocation /Torque Allocation ==
  T_req : Inport
  states : Inport  Port=2
  maxMotorTorque : Inport  Port=3
  Mz_ref : Inport  Port=4
  Mux1 : Mux  Inputs=3
  Mz : Scope
      settings: ShowLegends=on  TimeRange=24.149  YMin=-1  YMax=1.5  SaveName=ScopeData54
  Ti_max : Scope
      settings: ShowLegends=on  TimeRange=1.803977272727272  YMin=0  YMax=17  SaveName=ScopeData25
  TorqueAllocation : MATLAB Function  TreatAsAtomicUnit=on
  Ti_lim : Outport
  Mz_error : Outport  Port=2
  wires:
  T_req/1 -> TorqueAllocation/1(T_req)
  states/1 -> TorqueAllocation/2(states)
  TorqueAllocation/1(Ti_lim) -> Ti_lim/1
  Mz_ref/1 -> Mux1/3, TorqueAllocation/4(Mz_ref)  "Mz_ref"
  TorqueAllocation/2(Ti_max) -> Ti_max/1
  TorqueAllocation/3(Mz_error) -> Mux1/1, Mz_error/1  "Mz_error"
  TorqueAllocation/4(Mz_allocated) -> Mux1/2  "Mz_all"
  Mux1/1 -> Mz/1
  maxMotorTorque/1 -> TorqueAllocation/3(maxMotorTorque)

== system TV2016/CarMaker/IPG Vehicle/CarAndTrailer/CarAndTrailerUpd/CreateBus Brake.IF.In ==
  In : Inport
  BusCreator : BusCreator  Inputs=9
  Demux : Demux  Outputs=9
  Out : Outport
  wires:
  Demux/9 -> BusCreator/9  "Brake IF Trq_Reg RR"
  Demux/8 -> BusCreator/8  "Brake IF Trq_Reg RL"
  Demux/7 -> BusCreator/7  "Brake IF Trq_Reg FR"
  Demux/6 -> BusCreator/6  "Brake IF Trq_Reg FL"
  Demux/5 -> BusCreator/5  "Brake IF Trq_Reg_max RR"
  Demux/4 -> BusCreator/4  "Brake IF Trq_Reg_max RL"
  Demux/3 -> BusCreator/3  "Brake IF Trq_Reg_max FR"
  Demux/2 -> BusCreator/2  "Brake IF Trq_Reg_max FL"
  Demux/1 -> BusCreator/1  "Brake IF T_env"
  BusCreator/1 -> Out/1
  In/1 -> Demux/1

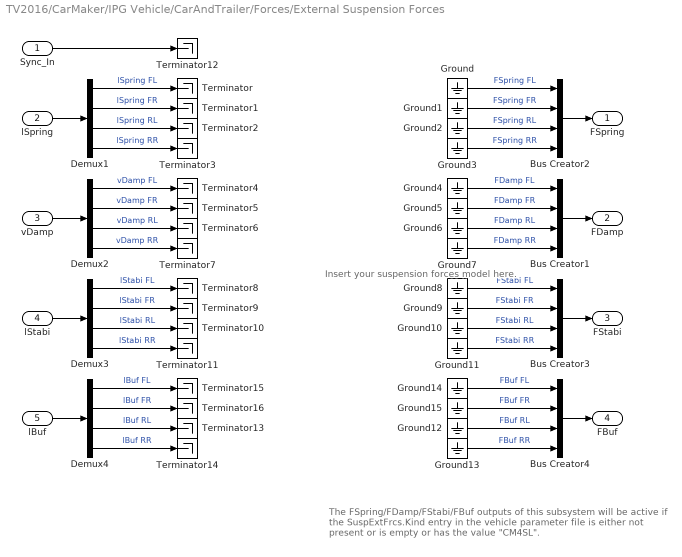
== system TV2016/CarMaker/IPG Vehicle/CarAndTrailer/Forces/External Suspension Forces ==
  note: The FSpring/FDamp/FStabi/FBuf outputs of this subsystem will be
      | active if the SuspExtFrcs.Kind entry in the vehicle parameter file
      | is either not present or is empty or has the value "CM4SL".
  note: Insert your suspension forces model here.
  Sync_In : Inport
  lSpring : Inport  Port=2
  vDamp : Inport  Port=3
  lStabi : Inport  Port=4
  lBuf : Inport  Port=5
  Bus Creator{1..4} (4 alike) : BusCreator
  Demux{1..4} (4 alike) : Demux
  Ground{,1..15} (16 alike) : Ground
  Terminator{,1..16} (17 alike) : Terminator
  FSpring : Outport
  FDamp : Outport  Port=2
  FStabi : Outport  Port=3
  FBuf : Outport  Port=4
  wires:
  lBuf/1 -> Demux4/1
  Demux4/1 -> Terminator15/1  "lBuf FL"
  Demux4/2 -> Terminator16/1  "lBuf FR"
  Demux4/3 -> Terminator13/1  "lBuf RL"
  Demux4/4 -> Terminator14/1  "lBuf RR"
  Ground14/1 -> Bus Creator4/1  "FBuf FL"
  Ground15/1 -> Bus Creator4/2  "FBuf FR"
  Ground12/1 -> Bus Creator4/3  "FBuf RL"
  Ground13/1 -> Bus Creator4/4  "FBuf RR"
  Bus Creator4/1 -> FBuf/1
  Sync_In/1 -> Terminator12/1
  lSpring/1 -> Demux1/1
  vDamp/1 -> Demux2/1
  lStabi/1 -> Demux3/1
  Demux3/1 -> Terminator8/1  "lStabi FL"
  Demux3/2 -> Terminator9/1  "lStabi FR"
  Demux3/3 -> Terminator10/1  "lStabi RL"
  Demux3/4 -> Terminator11/1  "lStabi RR"
  Demux1/1 -> Terminator/1  "lSpring FL"
  Demux1/2 -> Terminator1/1  "lSpring FR"
  Demux1/3 -> Terminator2/1  "lSpring RL"
  Demux1/4 -> Terminator3/1  "lSpring RR"
  Demux2/1 -> Terminator4/1  "vDamp FL"
  Demux2/2 -> Terminator5/1  "vDamp FR"
  Demux2/3 -> Terminator6/1  "vDamp RL"
  Demux2/4 -> Terminator7/1  "vDamp RR"
  Bus Creator2/1 -> FSpring/1
  Ground/1 -> Bus Creator2/1  "FSpring FL"
  Ground1/1 -> Bus Creator2/2  "FSpring FR"
  Ground2/1 -> Bus Creator2/3  "FSpring RL"
  Ground3/1 -> Bus Creator2/4  "FSpring RR"
  Ground4/1 -> Bus Creator1/1  "FDamp FL"
  Ground5/1 -> Bus Creator1/2  "FDamp FR"
  Ground6/1 -> Bus Creator1/3  "FDamp RL"
  Ground7/1 -> Bus Creator1/4  "FDamp RR"
  Bus Creator1/1 -> FDamp/1
  Ground8/1 -> Bus Creator3/1  "FStabi FL"
  Ground9/1 -> Bus Creator3/2  "FStabi FR"
  Ground10/1 -> Bus Creator3/3  "FStabi RL"
  Ground11/1 -> Bus Creator3/4  "FStabi RR"
  Bus Creator3/1 -> FStabi/1

== system TV2016/CarMaker/IPG Vehicle/CarAndTrailer/Forces/Tires ==
  note: The TireXX_Out signals will only be used if FileIdent is "CarMaker-Tire-CM4SL" in the tire parameter file!
      | An example parameter file can be found in Data/Tire/DT_CM4SL_UserTire.
  TireFL_In : Inport
  TireFR_In : Inport  Port=2
  TireRL_In : Inport  Port=3
  TireRR_In : Inport  Port=4
  Sync_In : Inport  Port=5
  Bus Creator{1..4} (4 alike) : BusCreator  Inputs=11
  Demux{1..3,8} (4 alike) : Demux  Outputs=7
  TireFL : Subsystem
  TireFR : Subsystem
  TireRL : Subsystem
  TireRR : Subsystem
  TireFL_Out : Outport
  TireFR_Out : Outport  Port=2
  TireRL_Out : Outport  Port=3
  TireRR_Out : Outport  Port=4
  wires:
  Sync_In/1 -> TireRR/1(Sync_In), TireRL/1(Sync_In), TireFR/1(Sync_In), TireFL/1(Sync_In)
  Bus Creator4/1 -> TireRR_Out/1
  Bus Creator2/1 -> TireRL_Out/1
  Bus Creator1/1 -> TireFR_Out/1
  Demux3/5 -> TireRR/6(Rim_turnv)  "Tire_In Rim_turnv"
  Demux3/4 -> TireRR/5(Rim_rotv)  "Tire_In Rim_rotv"
  Demux3/1 -> TireRR/2(Load)  "Tire_In Load"
  Demux3/7 -> TireRR/8(muRoad)  "Tire_In mu"
  Demux3/6 -> TireRR/7(InclinAngle)  "Tire_In Camber"
  Demux3/2 -> TireRR/3(vxtrans)  "Tire_In vxtrans"
  Demux3/3 -> TireRR/4(vytrans)  "Tire_In vytrans"
  TireRR/11(AlignTrq) -> Bus Creator4/11  "Tire_Out AlignTrq"
  TireRR/10(RollResist) -> Bus Creator4/10  "Tire_Out RollResist"
  TireRR/9(OverturnTrq) -> Bus Creator4/9  "Tire_Out OverturnTrq"
  TireRR/8(LoadFrc) -> Bus Creator4/8  "Tire_Out LoadFrc"
  TireRR/7(SideFrc) -> Bus Creator4/7  "Tire_Out SideFrc"
  TireRR/6(LongFrc) -> Bus Creator4/6  "Tire_Out LongFrc"
  TireRR/5(vBelt) -> Bus Creator4/5  "Tire_Out vBelt"
  TireRR/4(rBelt_eff) -> Bus Creator4/4  "Tire_Out rBelt_eff"
  TireRR/3(TurnSlp) -> Bus Creator4/3  "Tire_Out TurnSlp"
  TireRR/1(Slp) -> Bus Creator4/1  "Tire_Out Slp"
  TireRR/2(Alpha) -> Bus Creator4/2  "Tire_Out Alpha"
  Demux2/5 -> TireRL/6(Rim_turnv)  "Tire_In Rim_turnv"
  Demux2/4 -> TireRL/5(Rim_rotv)  "Tire_In Rim_rotv"
  Demux2/1 -> TireRL/2(Load)  "Tire_In Load"
  Demux2/7 -> TireRL/8(muRoad)  "Tire_In mu"
  Demux2/6 -> TireRL/7(InclinAngle)  "Tire_In Camber"
  Demux2/2 -> TireRL/3(vxtrans)  "Tire_In vxtrans"
  Demux2/3 -> TireRL/4(vytrans)  "Tire_In vytrans"
  TireRL/11(AlignTrq) -> Bus Creator2/11  "Tire_Out AlignTrq"
  TireRL/10(RollResist) -> Bus Creator2/10  "Tire_Out RollResist"
  TireRL/9(OverturnTrq) -> Bus Creator2/9  "Tire_Out OverturnTrq"
  TireRL/8(LoadFrc) -> Bus Creator2/8  "Tire_Out LoadFrc"
  TireRL/7(SideFrc) -> Bus Creator2/7  "Tire_Out SideFrc"
  TireRL/6(LongFrc) -> Bus Creator2/6  "Tire_Out LongFrc"
  TireRL/5(vBelt) -> Bus Creator2/5  "Tire_Out vBelt"
  TireRL/4(rBelt_eff) -> Bus Creator2/4  "Tire_Out rBelt_eff"
  TireRL/3(TurnSlp) -> Bus Creator2/3  "Tire_Out TurnSlp"
  TireRL/1(Slp) -> Bus Creator2/1  "Tire_Out Slp"
  TireRL/2(Alpha) -> Bus Creator2/2  "Tire_Out Alpha"
  Demux1/5 -> TireFR/6(Rim_turnv)  "Tire_In Rim_turnv"
  Demux1/4 -> TireFR/5(Rim_rotv)  "Tire_In Rim_rotv"
  Demux1/1 -> TireFR/2(Load)  "Tire_In Load"
  Demux1/7 -> TireFR/8(muRoad)  "Tire_In mu"
  Demux1/6 -> TireFR/7(InclinAngle)  "Tire_In Camber"
  Demux1/2 -> TireFR/3(vxtrans)  "Tire_In vxtrans"
  Demux1/3 -> TireFR/4(vytrans)  "Tire_In vytrans"
  TireFR/11(AlignTrq) -> Bus Creator1/11  "Tire_Out AlignTrq"
  TireFR/10(RollResist) -> Bus Creator1/10  "Tire_Out RollResist"
  TireFR/9(OverturnTrq) -> Bus Creator1/9  "Tire_Out OverturnTrq"
  TireFR/8(LoadFrc) -> Bus Creator1/8  "Tire_Out LoadFrc"
  TireFR/7(SideFrc) -> Bus Creator1/7  "Tire_Out SideFrc"
  TireFR/6(LongFrc) -> Bus Creator1/6  "Tire_Out LongFrc"
  TireFR/5(vBelt) -> Bus Creator1/5  "Tire_Out vBelt"
  TireFR/4(rBelt_eff) -> Bus Creator1/4  "Tire_Out rBelt_eff"
  TireFR/3(TurnSlp) -> Bus Creator1/3  "Tire_Out TurnSlp"
  TireFR/1(Slp) -> Bus Creator1/1  "Tire_Out Slp"
  TireFR/2(Alpha) -> Bus Creator1/2  "Tire_Out Alpha"
  Demux8/5 -> TireFL/6(Rim_turnv)  "Tire_In Rim_turnv"
  Demux8/4 -> TireFL/5(Rim_rotv)  "Tire_In Rim_rotv"
  TireFL_In/1 -> Demux8/1
  Demux8/1 -> TireFL/2(Load)  "Tire_In Load"
  Demux8/7 -> TireFL/8(muRoad)  "Tire_In mu"
  Demux8/6 -> TireFL/7(InclinAngle)  "Tire_In Camber"
  Demux8/2 -> TireFL/3(vxtrans)  "Tire_In vxtrans"
  Demux8/3 -> TireFL/4(vytrans)  "Tire_In vytrans"
  TireFL/11(AlignTrq) -> Bus Creator3/11  "Tire_Out AlignTrq"
  TireFL/10(RollResist) -> Bus Creator3/10  "Tire_Out RollResist"
  TireFL/9(OverturnTrq) -> Bus Creator3/9  "Tire_Out OverturnTrq"
  TireFL/8(LoadFrc) -> Bus Creator3/8  "Tire_Out LoadFrc"
  TireFL/7(SideFrc) -> Bus Creator3/7  "Tire_Out SideFrc"
  TireFL/6(LongFrc) -> Bus Creator3/6  "Tire_Out LongFrc"
  TireFL/5(vBelt) -> Bus Creator3/5  "Tire_Out vBelt"
  TireFL/4(rBelt_eff) -> Bus Creator3/4  "Tire_Out rBelt_eff"
  TireFL/3(TurnSlp) -> Bus Creator3/3  "Tire_Out TurnSlp"
  TireFL/1(Slp) -> Bus Creator3/1  "Tire_Out Slp"
  TireFL/2(Alpha) -> Bus Creator3/2  "Tire_Out Alpha"
  Bus Creator3/1 -> TireFL_Out/1
  TireFR_In/1 -> Demux1/1
  TireRL_In/1 -> Demux2/1
  TireRR_In/1 -> Demux3/1

== system TV2016/CarMaker/IPG Vehicle/CarAndTrailer/Forces/Vehicle Forces ==
  Sync_In : Inport
  Bus Creator1 : BusCreator  Inputs=12
  Bus Creator5 : BusCreator  Inputs=13
  Bus Creator8 : BusCreator  Inputs=16
  Demux : Demux  Outputs=16
  Demux1 : Demux  Outputs=12
  Demux5 : Demux  Outputs=13
  Forces : S-Function  FunctionName=CM_Sfun  Parameters='Forces'
  Sync_Out : Outport
  Car.Virtual : Outport  Port=2
  Car.Aero : Outport  Port=3
  Car.Load : Outport  Port=4
  wires:
  Demux/16 -> Bus Creator8/16  "Car Load_3 tz"
  Demux/15 -> Bus Creator8/15  "Car Load_3 ty"
  Demux/14 -> Bus Creator8/14  "Car Load_3 tx"
  Demux/13 -> Bus Creator8/13  "Car Load_3 mass"
  Demux1/12 -> Bus Creator1/12  "Car Virtual Trq_0 z"
  Demux1/11 -> Bus Creator1/11  "Car Virtual Trq_0 y"
  Demux1/10 -> Bus Creator1/10  "Car Virtual Trq_0 x"
  Demux1/9 -> Bus Creator1/9  "Car Virtual Trq_1 z"
  Demux1/8 -> Bus Creator1/8  "Car Virtual Trq_1 y"
  Demux1/7 -> Bus Creator1/7  "Car Virtual Trq_1 x"
  Demux1/6 -> Bus Creator1/6  "Car Virtual Frc_0 z"
  Demux1/5 -> Bus Creator1/5  "Car Virtual Frc_0 y"
  Demux1/4 -> Bus Creator1/4  "Car Virtual Frc_0 x"
  Sync_In/1 -> Forces/1
  Forces/1 -> Sync_Out/1
  Bus Creator5/1 -> Car.Aero/1
  Demux1/1 -> Bus Creator1/1  "Car Virtual Frc_1 x"
  Demux1/2 -> Bus Creator1/2  "Car Virtual Frc_1 y"
  Demux1/3 -> Bus Creator1/3  "Car Virtual Frc_1 z"
  Forces/3 -> Demux5/1
  Forces/2 -> Demux1/1
  Bus Creator1/1 -> Car.Virtual/1
  Bus Creator8/1 -> Car.Load/1
  Demux/1 -> Bus Creator8/1  "Car Load_0 mass"
  Demux/2 -> Bus Creator8/2  "Car Load_0 tx"
  Demux/3 -> Bus Creator8/3  "Car Load_0 ty"
  Demux/4 -> Bus Creator8/4  "Car Load_0 tz"
  Demux/5 -> Bus Creator8/5  "Car Load_1 mass"
  Demux/6 -> Bus Creator8/6  "Car Load_1 tx"
  Demux/7 -> Bus Creator8/7  "Car Load_1 ty"
  Demux/8 -> Bus Creator8/8  "Car Load_1 tz"
  Demux/9 -> Bus Creator8/9  "Car Load_2 mass"
  Demux/10 -> Bus Creator8/10  "Car Load_2 tx"
  Demux/11 -> Bus Creator8/11  "Car Load_2 ty"
  Demux/12 -> Bus Creator8/12  "Car Load_2 tz"
  Forces/4 -> Demux/1
  Demux5/11 -> Bus Creator5/11  "car Aero Trq_1 x"
  Demux5/12 -> Bus Creator5/12  "car Aero Trq_1 y"
  Demux5/13 -> Bus Creator5/13  "car Aero Trq_1 z"
  Demux5/10 -> Bus Creator5/10  "car Aero Frc_1 z"
  Demux5/9 -> Bus Creator5/9  "car Aero Frc_1 y"
  Demux5/8 -> Bus Creator5/8  "car Aero Frc_1 x"
  Demux5/1 -> Bus Creator5/1  "Vehicle sRoadAero"
  Demux5/2 -> Bus Creator5/2  "Vehicle Wind_vel_0 x"
  Demux5/3 -> Bus Creator5/3  "Vehicle Wind_vel_0 y"
  Demux5/4 -> Bus Creator5/4  "Vehicle Wind_vel_0 z"
  Demux5/5 -> Bus Creator5/5  "car Aero vRes_1 x"
  Demux5/6 -> Bus Creator5/6  "car Aero vRes_1 y"
  Demux5/7 -> Bus Creator5/7  "car Aero vRes_1 z"

== system TV2016/CarMaker/IPG Vehicle/CarAndTrailer/Trailer/CreateBus Car.Hitch.FrcTrq ==
  In1 : Inport
  Bus Creator7 : BusCreator  Inputs=6
  Demux7 : Demux  Outputs=6
  Car.Hitch.FrcTrq : Outport
  wires:
  In1/1 -> Demux7/1
  Bus Creator7/1 -> Car.Hitch.FrcTrq/1
  Demux7/6 -> Bus Creator7/6  "Car Hitch Trq2Car z"
  Demux7/5 -> Bus Creator7/5  "Car Hitch Trq2Car y"
  Demux7/4 -> Bus Creator7/4  "Car Hitch Trq2Car x"
  Demux7/3 -> Bus Creator7/3  "Car Hitch Frc2Car z"
  Demux7/2 -> Bus Creator7/2  "Car Hitch Frc2Car y"
  Demux7/1 -> Bus Creator7/1  "Car Hitch Frc2Car x"

== system TV2016/CarMaker/IPG Vehicle/CarAndTrailer/Trailer/CreateBus Vhcl.Motion ==
  In1 : Inport
  Demux1 : Demux  Outputs=16
  Mux1 : Mux  Inputs=16
  Out1 : Outport
  wires:
  Demux1/1 -> Mux1/1  "Vhcl v"
  Demux1/2 -> Mux1/2  "Vhcl Distance"
  Demux1/3 -> Mux1/3  "Vhcl sRoad"
  Demux1/4 -> Mux1/4  "Vhcl sRoadAero"
  Demux1/5 -> Mux1/5  "Vhcl Hitch_Pos x"
  Demux1/6 -> Mux1/6  "Vhcl Hitch_Pos y"
  Demux1/7 -> Mux1/7  "Vhcl Hitch_Pos z"
  Demux1/8 -> Mux1/8  "Vhcl Roll"
  Demux1/9 -> Mux1/9  "Vhcl RollVel"
  Demux1/10 -> Mux1/10  "Vhcl RollAcc"
  Demux1/11 -> Mux1/11  "Vhcl Pitch"
  Demux1/12 -> Mux1/12  "Vhcl PitchVel"
  Demux1/13 -> Mux1/13  "Vhcl PitchAcc"
  Demux1/14 -> Mux1/14  "Vhcl Yaw"
  Demux1/15 -> Mux1/15  "Vhcl YawRate"
  Demux1/16 -> Mux1/16  "Vhcl YawAcc"
  In1/1 -> Demux1/1
  Mux1/1 -> Out1/1

== system TV2016/CarMaker/IPG Vehicle/CarAndTrailer/Trailer/CreateBus Vhcl.PoI ==
  In1 : Inport
  Bus Creator3 : BusCreator  Inputs=18
  Demux3 : Demux  Outputs=18
  Out1 : Outport
  wires:
  Demux3/18 -> Bus Creator3/18  "Vhcl PoI_GCS Elev"
  Demux3/17 -> Bus Creator3/17  "Vhcl PoI_GCS Lat"
  Demux3/16 -> Bus Creator3/16  "Vhcl PoI_GCS Long"
  Demux3/15 -> Bus Creator3/15  "Vhcl PoI_Acc_1 z"
  Demux3/14 -> Bus Creator3/14  "Vhcl PoI_Acc_1 y"
  Demux3/13 -> Bus Creator3/13  "Vhcl PoI_Acc_1 x"
  Demux3/12 -> Bus Creator3/12  "Vhcl PoI_Vel_1 z"
  Demux3/11 -> Bus Creator3/11  "Vhcl PoI_Vel_1 y"
  Demux3/10 -> Bus Creator3/10  "Vhcl PoI_Vel_1 x"
  Demux3/9 -> Bus Creator3/9  "Vhcl PoI_Acc z"
  Demux3/8 -> Bus Creator3/8  "Vhcl PoI_Acc y"
  Demux3/7 -> Bus Creator3/7  "Vhcl PoI_Acc x"
  Demux3/6 -> Bus Creator3/6  "Vhcl PoI_Vel z"
  Demux3/5 -> Bus Creator3/5  "Vhcl PoI_Vel y"
  Demux3/4 -> Bus Creator3/4  "Vhcl PoI_Vel x"
  Demux3/3 -> Bus Creator3/3  "Vhcl PoI_Pos z"
  Demux3/2 -> Bus Creator3/2  "Vhcl PoI_Pos y"
  In1/1 -> Demux3/1
  Bus Creator3/1 -> Out1/1
  Demux3/1 -> Bus Creator3/1  "Vhcl PoI_Pos x"

== system TV2016/CarMaker/IPG Vehicle/CarAndTrailer/Trailer/CreateBus Vhcl.Steering ==
  In1 : Inport
  Bus Creator3 : BusCreator
  Demux : Demux
  Out1 : Outport
  wires:
  Bus Creator3/1 -> Out1/1
  Demux/1 -> Bus Creator3/1  "Vhcl Steering Ang"
  Demux/3 -> Bus Creator3/3  "Vhcl Steering AngAcc"
  Demux/2 -> Bus Creator3/2  "Vhcl Steering AngVel"
  Demux/4 -> Bus Creator3/4  "Vhcl Steering Trq"
  In1/1 -> Demux/1

== system TV2016/CarMaker/IPG Vehicle/CarAndTrailer/Trailer/CreateBus Vhcl.Wheel.FL ==
  In1 : Inport
  Bus Creator3 : BusCreator  Inputs=14
  Demux3 : Demux  Outputs=14
  Out1 : Outport
  wires:
  Demux3/14 -> Bus Creator3/14  "Vhcl Wheel FL Trq_WhlBearing"
  Demux3/13 -> Bus Creator3/13  "Vhcl Wheel FL Trq_T2W"
  Demux3/12 -> Bus Creator3/12  "Vhcl Wheel FL SideSlip"
  Demux3/11 -> Bus Creator3/11  "Vhcl Wheel FL LongSlip"
  Demux3/10 -> Bus Creator3/10  "Vhcl Wheel FL vBelt"
  Demux3/9 -> Bus Creator3/9  "Vhcl Wheel FL Fz"
  Demux3/8 -> Bus Creator3/8  "Vhcl Wheel FL Fy"
  Demux3/7 -> Bus Creator3/7  "Vhcl Wheel FL Fx"
  Demux3/6 -> Bus Creator3/6  "Vhcl Wheel FL r_zxy z"
  Demux3/5 -> Bus Creator3/5  "Vhcl Wheel FL r_zxy y"
  Demux3/4 -> Bus Creator3/4  "Vhcl Wheel FL r_zxy x"
  Demux3/3 -> Bus Creator3/3  "Vhcl Wheel FL t z"
  Demux3/2 -> Bus Creator3/2  "Vhcl Wheel FL t y"
  In1/1 -> Demux3/1
  Bus Creator3/1 -> Out1/1
  Demux3/1 -> Bus Creator3/1  "Vhcl Wheel FL t x"

== system TV2016/CarMaker/IPG Vehicle/CarAndTrailer/Trailer/CreateBus Vhcl.Wheel.FR ==
  In1 : Inport
  Bus Creator3 : BusCreator  Inputs=14
  Demux3 : Demux  Outputs=14
  Out1 : Outport
  wires:
  Demux3/14 -> Bus Creator3/14  "Vhcl Wheel FR Trq_WhlBearing"
  Demux3/13 -> Bus Creator3/13  "Vhcl Wheel FR Trq_T2W"
  Demux3/12 -> Bus Creator3/12  "Vhcl Wheel FR SideSlip"
  Demux3/11 -> Bus Creator3/11  "Vhcl Wheel FR LongSlip"
  Demux3/10 -> Bus Creator3/10  "Vhcl Wheel FR vBelt"
  Demux3/9 -> Bus Creator3/9  "Vhcl Wheel FR Fz"
  Demux3/8 -> Bus Creator3/8  "Vhcl Wheel FR Fy"
  Demux3/7 -> Bus Creator3/7  "Vhcl Wheel FR Fx"
  Demux3/6 -> Bus Creator3/6  "Vhcl Wheel FR r_zxy z"
  Demux3/5 -> Bus Creator3/5  "Vhcl Wheel FR r_zxy y"
  Demux3/4 -> Bus Creator3/4  "Vhcl Wheel FR r_zxy x"
  Demux3/3 -> Bus Creator3/3  "Vhcl Wheel FR t z"
  Demux3/2 -> Bus Creator3/2  "Vhcl Wheel FR t y"
  In1/1 -> Demux3/1
  Bus Creator3/1 -> Out1/1
  Demux3/1 -> Bus Creator3/1  "Vhcl Wheel FR t x"

== system TV2016/CarMaker/IPG Vehicle/CarAndTrailer/Trailer/CreateBus Vhcl.Wheel.RL ==
  In1 : Inport
  Bus Creator3 : BusCreator  Inputs=14
  Demux3 : Demux  Outputs=14
  Out1 : Outport
  wires:
  Demux3/14 -> Bus Creator3/14  "Vhcl Wheel RL Trq_WhlBearing"
  Demux3/13 -> Bus Creator3/13  "Vhcl Wheel RL Trq_T2W"
  Demux3/12 -> Bus Creator3/12  "Vhcl Wheel RL SideSlip"
  Demux3/11 -> Bus Creator3/11  "Vhcl Wheel RL LongSlip"
  Demux3/10 -> Bus Creator3/10  "Vhcl Wheel RL vBelt"
  Demux3/9 -> Bus Creator3/9  "Vhcl Wheel RL Fz"
  Demux3/8 -> Bus Creator3/8  "Vhcl Wheel RL Fy"
  Demux3/7 -> Bus Creator3/7  "Vhcl Wheel RL Fx"
  Demux3/6 -> Bus Creator3/6  "Vhcl Wheel RL r_zxy z"
  Demux3/5 -> Bus Creator3/5  "Vhcl Wheel RL r_zxy y"
  Demux3/4 -> Bus Creator3/4  "Vhcl Wheel RL r_zxy x"
  Demux3/3 -> Bus Creator3/3  "Vhcl Wheel RL t z"
  Demux3/2 -> Bus Creator3/2  "Vhcl Wheel RL t y"
  In1/1 -> Demux3/1
  Bus Creator3/1 -> Out1/1
  Demux3/1 -> Bus Creator3/1  "Vhcl Wheel RL t x"
